simulink model "ECU_Auxiliaries_Signal_Coordinator_RefMdl"  (R2016b)
settings: Solver=FixedStepDiscrete  StartTime=0.0  StopTime=inf  RelTol=1e-3  EnableMultiTasking=on
settings Model: Creator=djuenema  LastModifiedBy=djuenema
settings DataIOCC: SaveFormat=StructureWithTime  SaveOutput=off  DSMLogging=off  VisualizeSimOutput=off  SaveTime=off  SignalLoggingName=Results
settings OptimizationCC: BlockReduction=off  ConditionallyExecuteInputs=off  LifeSpan=inf
settings DebuggingCC: AllowSymbolicDim=off  SFUnexpectedBacktrackingDiag=warning  SFNoUnconditionalDefaultTransitionDiag=warning  SFExecutionAtInitializationDiag=none
settings ModelReferenceCC: PropagateSignalLabelsOutOfModel=off
settings GRTTargetCC: TargetLangStandard=C89/C90 (ANSI)
settings ConfigComp: CovMetricSettings=dw  CovHtmlReporting=on  CovSaveCumulativeToWorkspaceVar=on  CovSaveSingleToWorkspaceVar=on  CovExternalEMLEnable=off

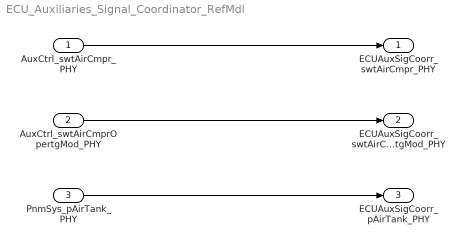
== system ECU_Auxiliaries_Signal_Coordinator_RefMdl ==
  AuxCtrl_swtAirCmpr_PHY : Inport
  AuxCtrl_swtAirCmprOpertgMod_PHY : Inport  Port=2
  PnmSys_pAirTank_PHY : Inport  Port=3
  ECUAuxSigCoorr_swtAirCmpr_PHY : Outport
  ECUAuxSigCoorr_swtAirCmprOpertgMod_PHY : Outport  Port=2
  ECUAuxSigCoorr_pAirTank_PHY : Outport  Port=3
  wires:
  PnmSys_pAirTank_PHY/1 -> ECUAuxSigCoorr_pAirTank_PHY/1
  AuxCtrl_swtAirCmpr_PHY/1 -> ECUAuxSigCoorr_swtAirCmpr_PHY/1
  AuxCtrl_swtAirCmprOpertgMod_PHY/1 -> ECUAuxSigCoorr_swtAirCmprOpertgMod_PHY/1
